simulink model "modelo_armonicos_60hz"  (R2025b)
settings: Solver=FixedStepDiscrete  StartTime=0.0  StopTime=0.1  FixedStep=0.0001  RelTol=1e-3
settings Model: Creator=johnd  LastModifiedBy=johnd

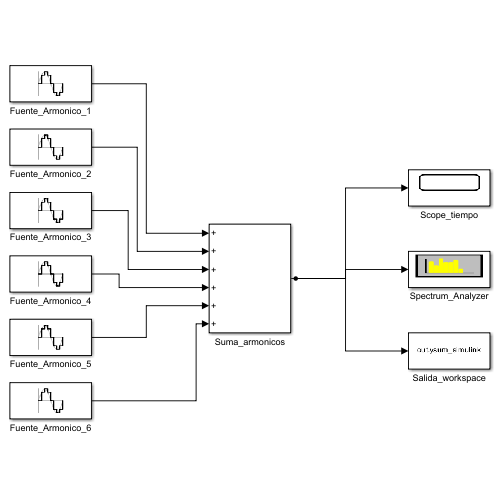
[thumbnail: Simulink's stored preview of the top-level diagram]
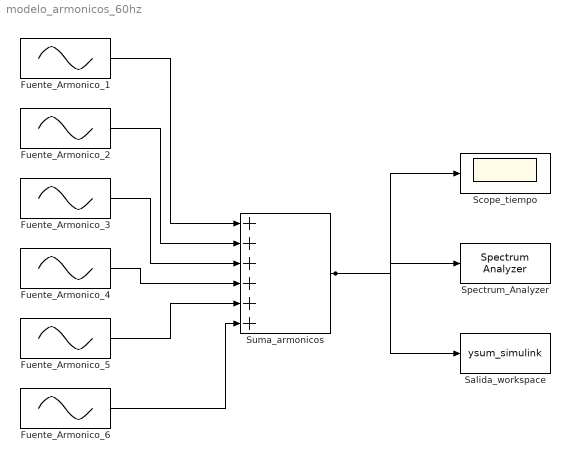
== system modelo_armonicos_60hz ==
  Fuente_Armonico_1 : Sin  Amplitude=120  Frequency=376.9911  SampleTime=0.0001
  Fuente_Armonico_2 : Sin  Amplitude=60  Frequency=753.9822  SampleTime=0.0001
  Fuente_Armonico_3 : Sin  Amplitude=40  Frequency=1130.9734  SampleTime=0.0001
  Fuente_Armonico_4 : Sin  Amplitude=30  Frequency=1507.9645  SampleTime=0.0001
  Fuente_Armonico_5 : Sin  Amplitude=24  Frequency=1884.9556  SampleTime=0.0001
  Fuente_Armonico_6 : Sin  Amplitude=20  Frequency=2261.9467  SampleTime=0.0001
  Salida_workspace : ToWorkspace  VariableName=ysum_simulink  SaveFormat=Structure With Time  SampleTime=-1
  Scope_tiempo : Scope
  Spectrum_Analyzer : SpectrumAnalyzer  WindowPosition=[240.000000,150.000000,800.000000,500.000000,]  Visible=on  ScopeFrameLocation=window  WindowInvariantSamplesPerUpdate=on  YLimits=[-132.618 87.6308]
  Suma_armonicos : Sum  Inputs=++++++
  wires:
  Fuente_Armonico_1/1 -> Suma_armonicos/1
  Fuente_Armonico_2/1 -> Suma_armonicos/2
  Fuente_Armonico_3/1 -> Suma_armonicos/3
  Fuente_Armonico_4/1 -> Suma_armonicos/4
  Fuente_Armonico_5/1 -> Suma_armonicos/5
  Fuente_Armonico_6/1 -> Suma_armonicos/6
  Suma_armonicos/1 -> Scope_tiempo/1, Spectrum_Analyzer/1, Salida_workspace/1
